simulink model "rtwdemo_clibsup"  (Simulink 6.0)
settings: Solver=FixedStepDiscrete  StartTime=0.0  StopTime=10.0  RelTol=1e-3
undefined symbols (not defined in the file or in its folder): magnitude
libraries: rtwdemowidgets x3
settings Model: Creator=The MathWorks Inc.  LastModifiedBy=batserve  ExtModeAutoUpdateStatusClock=off
settings DataIOCC: SaveOutput=off  SaveTime=off  SignalLoggingName=sigsOut
settings OptimizationCC: InlineParams=on  EnforceIntegerDowncast=off  StateBitsets=on  DataBitsets=on  UseTempVars=on
settings DebuggingCC: CheckExecutionContextPreStartOutputMsg=on  CheckExecutionContextRuntimeOutputMsg=on  SolverPrmCheckMsg=none
settings RTWCC: TLCOptions=-p0 -aWarnNonSaturatedBlocks=0  GenCodeOnly=on  GenerateReport=on  RTWVerbose=off  ProcessScript=grt_make_rtw_hook  LaunchReport=on
settings CodeAppCC: ForceParamTrailComments=on  PrefixModelToSubsysFcnNames=off

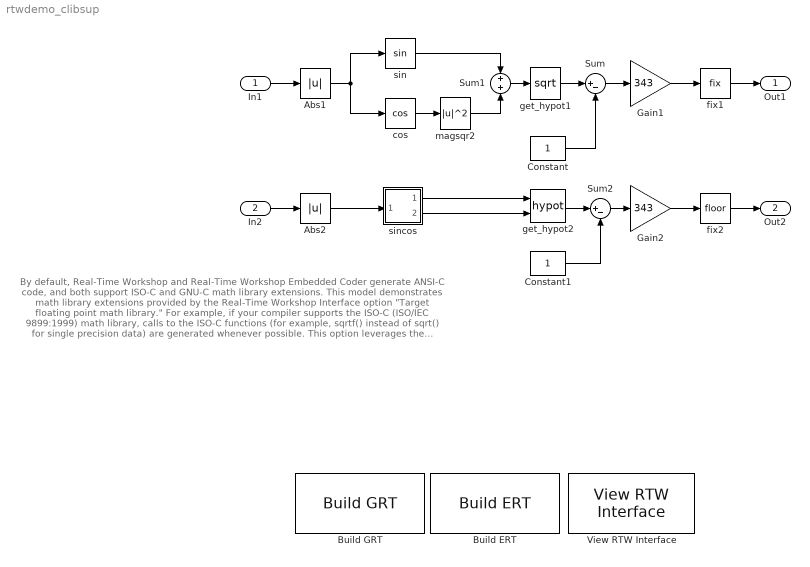
== system rtwdemo_clibsup ==
  note: By default, Real-Time Workshop and Real-Time Workshop Embedded Coder generate ANSI-C code, and
      | both support ISO-C and GNU-C math library extensions.  This model demonstrates math library
      | extensions provided by the Real-Time Workshop Interface option "Target floating point math
      | library."
      |
      | For example, if your compiler supports the ISO-C (ISO/IEC 9899:1999) math library, calls to
      | the ISO-C functions (for example, sqrtf() instead of sqrt() for single precision data) are
      | generated whenever possible.  This option leverages the performance your target compiler offers
      | over standard ANSI-C.
  In1 : Inport  Port=1  SampleTime=1  DataType=single  LatchInput=off
  In2 : Inport  Port=2  SampleTime=1  DataType=single  LatchInput=off
  Abs1 : Abs  SaturateOnIntegerOverflow=on
  Abs2 : Abs  SaturateOnIntegerOverflow=on
  Build ERT : rtwdemowidgets/Build ERT  attrib_overrides={'GenFloatMathFcnCalls'}
  Build GRT : rtwdemowidgets/Build GRT  attrib_overrides={'GenFloatMathFcnCalls'}
  Constant : Constant
  Constant1 : Constant
  Gain1 : Gain  Gain=343  SaturateOnIntegerOverflow=on
  Gain2 : Gain  Gain=343  SaturateOnIntegerOverflow=on
  Sum : Sum  Inputs=|+-  SaturateOnIntegerOverflow=on  InputSameDT=on
  Sum1 : Sum  SaturateOnIntegerOverflow=on  InputSameDT=on
  Sum2 : Sum  Inputs=|+-  SaturateOnIntegerOverflow=on  InputSameDT=on
  View RTW Interface : rtwdemowidgets/View RTW Interface
  cos : Trigonometry  Operator=cos
  fix1 : Rounding  Operator=fix
  fix2 : Rounding
  get_hypot1 : Math  Operator=sqrt  SaturateOnIntegerOverflow=on
  get_hypot2 : Math  Operator=hypot  SaturateOnIntegerOverflow=on
  magsqr2 : Math  Operator=magnitude^2  SaturateOnIntegerOverflow=on
  sin : Trigonometry
  sincos : Subsystem  PropExecContextAcrossSSBoundary=on
      mask Display: text(0.5,0.5,'sincos','horizontalAlignment','center')
  Out1 : Outport
  Out2 : Outport  Port=2
  wires:
  In1/1 -> Abs1/1
  sin/1 -> Sum1/1
  cos/1 -> magsqr2/1
  get_hypot1/1 -> Sum/1
  Abs1/1 -> sin/1, cos/1
  Constant/1 -> Sum/2
  Sum/1 -> Gain1/1
  Sum1/1 -> get_hypot1/1
  magsqr2/1 -> Sum1/2
  sincos/1(Out1) -> get_hypot2/1
  sincos/2(Out2) -> get_hypot2/2
  get_hypot2/1 -> Sum2/1
  Sum2/1 -> Gain2/1
  Constant1/1 -> Sum2/2
  In2/1 -> Abs2/1
  Abs2/1 -> sincos/1(In1)
  Gain1/1 -> fix1/1
  Gain2/1 -> fix2/1
  fix1/1 -> Out1/1
  fix2/1 -> Out2/1

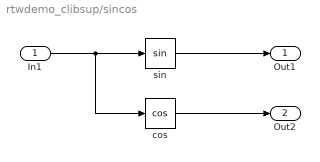
== system rtwdemo_clibsup/sincos ==
  In1 : Inport  Port=1  LatchInput=off
  cos : Trigonometry  Operator=cos
  sin : Trigonometry
  Out1 : Outport
  Out2 : Outport  Port=2
  wires:
  In1/1 -> sin/1, cos/1
  sin/1 -> Out1/1
  cos/1 -> Out2/1
